simulink model "twolink_sim"  (R2021b)
settings: Solver=VariableStepAuto  StartTime=0.0  StopTime=1  RelTol=1e-3
settings Model: Creator=Super  LastModifiedBy=Super
settings DataIOCC: ReturnWorkspaceOutputs=off

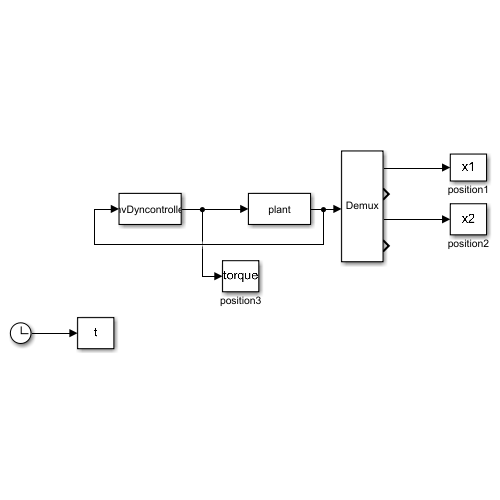
[thumbnail: Simulink's stored preview of the top-level diagram]
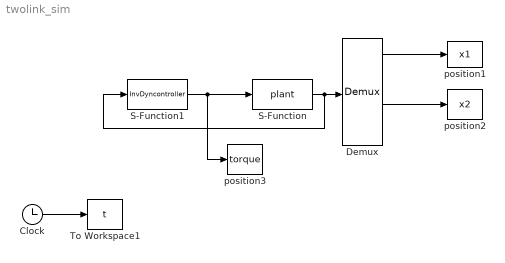
== system twolink_sim ==
  Clock : Clock
  Demux : Demux
      settings: DisplayOption=none
  S-Function : S-Function  FunctionName=plant  SFunctionDeploymentMode=off  EnableBusSupport=off
  S-Function1 : S-Function  FunctionName=InvDyncontroller  SFunctionDeploymentMode=off  EnableBusSupport=off
  To Workspace1 : ToWorkspace  VariableName=t  SampleTime=-1
  position1 : ToWorkspace  VariableName=x1  SampleTime=-1
  position2 : ToWorkspace  VariableName=x2  SampleTime=-1
  position3 : ToWorkspace  VariableName=torque  SampleTime=-1
  wires:
  S-Function1/1 -> position3/1, S-Function/1
  S-Function/1 -> S-Function1/1, Demux/1
  Clock/1 -> To Workspace1/1
  Demux/1 -> position1/1
  Demux/3 -> position2/1
